simulink model "simulacion_impulso_controlador"  (R2021a)
settings: Solver=VariableStepAuto  StartTime=0.0  StopTime=20.0  RelTol=1e-3
values from neighbouring files (symbols this model uses):
  K = -dlqr(modelo_ss_d.A, modelo_ss_d.B,Q,R)    [controlador.m]    (also in controlador_integral.m = -place(planta_seguimiento_ss_r_d.A , planta_seguimiento_ss_r; precompensacion.m = -place(modelo_ss_d.A , modelo_ss_d.B , plc_d); tp4_matlab.m = -place(modelo_ss_d.A , modelo_ss_d.B , plc_d))
  modelo_ss_d = c2d(modelo_ss,Ts)    [controlador.m]    (also in observador.m; precompensacion.m; tp4_matlab.m)
settings Model: Creator=nnobi  LastModifiedBy=nnobi

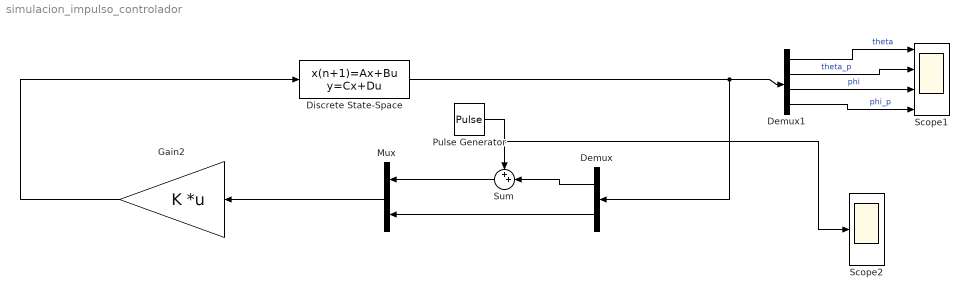
== system simulacion_impulso_controlador ==
  Demux : Demux  Outputs=[1 3]
  Demux1 : Demux
  Discrete State-Space : DiscreteStateSpace  A=modelo_ss_d.A  B=modelo_ss_d.B  C=[1 0 0 0; 0 1 0 0; 0 0 1 0; 0 0 0 1]  D=[0; 0; 0; 0]  SampleTime=0.01
  Gain2 : Gain  Gain=K  Multiplication=Matrix(K*u)
  Mux : Mux  Inputs=[1 3]
  Pulse Generator : DiscretePulseGenerator  PulseType=Time based  Amplitude=-0.9  Period=100  PulseWidth=0.1  PhaseDelay=1.24
  Scope1 : Scope  NumInputPorts=4
  Scope2 : Scope
  Sum : Sum  Inputs=++|
  wires:
  Gain2/1 -> Discrete State-Space/1
  Demux/2 -> Mux/2
  Mux/1 -> Gain2/1
  Discrete State-Space/1 -> Demux1/1, Demux/1
  Pulse Generator/1 -> Scope2/1, Sum/1
  Demux/1 -> Sum/2
  Sum/1 -> Mux/1
  Demux1/1 -> Scope1/1  "theta"
  Demux1/2 -> Scope1/2  "theta_p"
  Demux1/3 -> Scope1/3  "phi"
  Demux1/4 -> Scope1/4  "phi_p"
